simulink model "CL_NL_DH_GUIA"  (R2025b)
settings: Solver=ode4  StartTime=0.0  StopTime=200  FixedStep=Ts  RelTol=1e-3
values from neighbouring files (symbols this model uses):
  att_alt = 0    [guiagem_NL.m]
  h_ref0 = h0    (= 600)    [guiagem_NL.m]
  i = find([Plantas.Ve] == VT_missao & [Plantas.He] == 600, 1)    [guiagem_NL.m]
  K_bank_guia = 0.1975    [guiagem_NL.m]
  phi_max_guia = deg2rad(20)    [guiagem_NL.m]
  phi_psi = 0    [guiagem_NL.m]
  surfaces = 24    [guiagem_NL.m]
  U_trim = double(Plantas(i).Ue(1:4))    [guiagem_NL.m]
  VT_ref0 = VT_missao    [guiagem_NL.m]
  VT_Throttle = 1    [guiagem_NL.m]
  WPs = [ 256    0  600  15 ... (first row only)    [guiagem_NL.m]
undefined symbols (not defined in the file or in its folder): Plantas, R_accept
libraries: simulink_extras x10, simulink x1
settings Model: SimulationMode=accelerator  Creator=mirko  LastModifiedBy=mirko

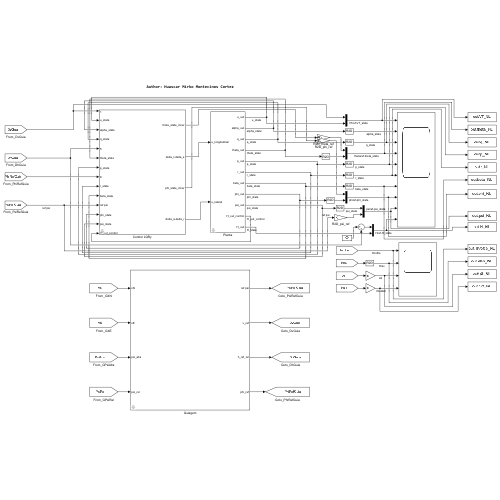
[thumbnail: Simulink's stored preview of the top-level diagram]
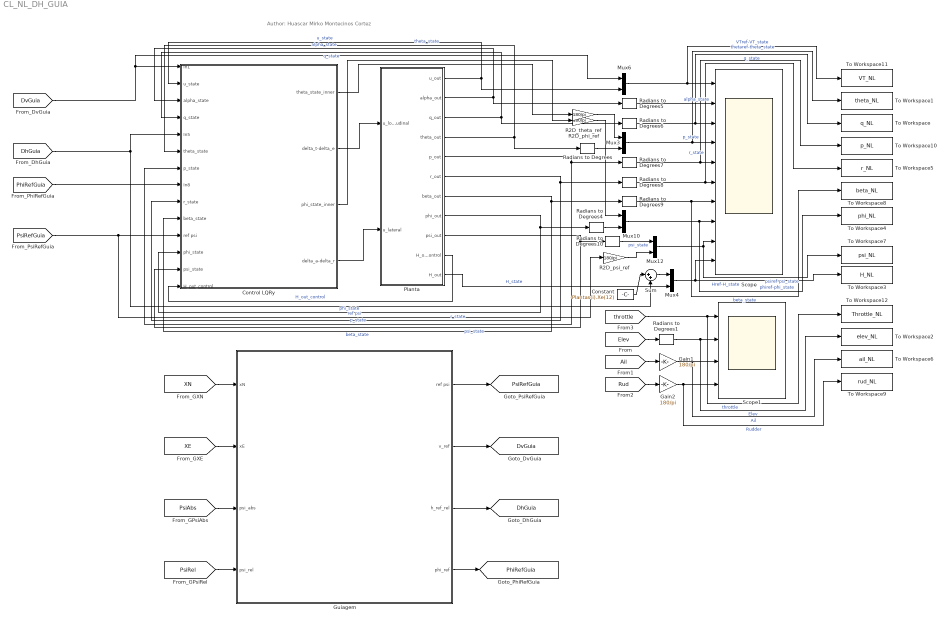
== system CL_NL_DH_GUIA ==
  note: Author: Huascar Mirko Montecinos Cortez
  Constant : Constant  Value=-Plantas(i).Xe(12)
  Control LQRy : Subsystem
  Gain1 : Gain  Gain=180/pi
  Gain2 : Gain  Gain=180/pi
  Guiagem : Subsystem
  Mux{3..4,6,10,12} (5 alike) : Mux  Inputs=2
  Planta : Subsystem
  R2D_phi_ref : Gain  Gain=180/pi
  R2D_psi_ref : Gain  Gain=180/pi
  R2D_theta_ref : Gain  Gain=180/pi
  Radians to Degrees{,1,4..10} (9 alike) : simulink_extras/Transformations/Radians to Degrees
  Scope : Scope  NumInputPorts=10
      settings: ActiveDisplayString=10  ActiveDisplayYMinimum=597.42662245797032  ActiveDisplayYMaximum=600.90765479327524
  Scope1 : Scope  NumInputPorts=4
      settings: ActiveDisplayString=4  ActiveDisplayYMinimum=-5.76866006164083  ActiveDisplayYMaximum=6.0116826932203384
  Sum : Sum  Inputs=|++
  To Workspace : ToWorkspace  VariableName=q_NL  SaveFormat=Structure With Time  SampleTime=-1
  To Workspace1 : ToWorkspace  VariableName=theta_NL  SaveFormat=Structure With Time  SampleTime=-1
  To Workspace10 : ToWorkspace  VariableName=p_NL  SaveFormat=Structure With Time  SampleTime=-1
  To Workspace11 : ToWorkspace  VariableName=VT_NL  SaveFormat=Structure With Time  SampleTime=-1
  To Workspace12 : ToWorkspace  VariableName=Throttle_NL  SaveFormat=Structure With Time  SampleTime=-1
  To Workspace2 : ToWorkspace  VariableName=elev_NL  SaveFormat=Structure With Time  SampleTime=-1
  To Workspace3 : ToWorkspace  VariableName=H_NL  SaveFormat=Structure With Time  SampleTime=-1
  To Workspace4 : ToWorkspace  VariableName=phi_NL  SaveFormat=Structure With Time  SampleTime=-1
  To Workspace5 : ToWorkspace  VariableName=r_NL  SaveFormat=Structure With Time  SampleTime=-1
  To Workspace6 : ToWorkspace  VariableName=ail_NL  SaveFormat=Structure With Time  SampleTime=-1
  To Workspace7 : ToWorkspace  VariableName=psi_NL  SaveFormat=Structure With Time  SampleTime=-1
  To Workspace8 : ToWorkspace  VariableName=beta_NL  SaveFormat=Structure With Time  SampleTime=-1
  To Workspace9 : ToWorkspace  VariableName=rud_NL  SaveFormat=Structure With Time  SampleTime=-1
  tag scope: DhGuia=global, DvGuia=global, PhiRefGuia=global, PsiRefGuia=global
  wires:
  Planta/1(u_out) -> Mux6/2, Control LQRy/2(u_state)  "u_state"
  Planta/2(alpha_out) -> Radians to Degrees5/1, Control LQRy/3(alpha_state)  "alpha_state"
  Planta/3(q_out) -> Radians to Degrees6/1, Control LQRy/4(q_state)  "q_state"
  Planta/4(theta_out) -> Radians to Degrees/1, Control LQRy/6(theta_state)  "theta_state"
  Planta/5(p_out) -> Control LQRy/7(p_state), Radians to Degrees7/1  "p_state"
  Planta/6(r_out) -> Radians to Degrees8/1, Control LQRy/9(r_state)  "r_state"
  Planta/7(beta_out) -> Control LQRy/10(beta_state), Radians to Degrees9/1  "beta_state"
  Planta/8(phi_out) -> Control LQRy/12(phi_state), Radians to Degrees4/1  "phi_state"
  Planta/9(psi_out) -> Control LQRy/13(psi_state), Radians to Degrees10/1  "psi_state"
  Mux3/1 -> To Workspace1/1, Scope/4  "thetaref-theta_state"
  Radians to Degrees/1 -> Mux3/2
  Mux4/1 -> Scope/10, To Workspace3/1  "Href-H_state"
  Constant/1 -> Sum/1
  Sum/1 -> Mux4/1
  Radians to Degrees1/1 -> Scope1/2, To Workspace2/1  "Elev"
  Gain1/1 -> Scope1/3, To Workspace6/1  "Ail"
  Gain2/1 -> Scope1/4, To Workspace9/1  "Rudder"
  [Elev] -> Radians to Degrees1/1
  [Ail] -> Gain1/1
  [Rud] -> Gain2/1
  [throttle] -> To Workspace12/1, Scope1/1  "throttle"
  Mux6/1 -> To Workspace11/1, Scope/1  "VTref-VT_state"
  Mux10/1 -> To Workspace4/1, Scope/8  "phiref-phi_state"
  Radians to Degrees4/1 -> Mux10/2
  Radians to Degrees5/1 -> Scope/2  "alpha_state"
  Radians to Degrees6/1 -> To Workspace/1, Scope/3  "q_state"
  Radians to Degrees7/1 -> To Workspace10/1, Scope/5  "p_state"
  Radians to Degrees8/1 -> Scope/6, To Workspace5/1  "r_state"
  Radians to Degrees9/1 -> Scope/7, To Workspace8/1  "beta_state"
  Mux12/1 -> To Workspace7/1, Scope/9  "psiref-psi_state"
  Planta/11(H_out) -> Mux4/2  "H_state"
  Radians to Degrees10/1 -> Mux12/1  "psi_state"
  [DhGuia] -> Sum/2, Control LQRy/5(In5)
  [DvGuia] -> Mux6/1, Control LQRy/1(In1)
  R2D_theta_ref/1 -> Mux3/1
  R2D_psi_ref/1 -> Mux12/2
  R2D_phi_ref/1 -> Mux10/1
  [PsiRefGuia] -> R2D_psi_ref/1, Control LQRy/11(ref psi)  "ref psi"
  [PhiRefGuia] -> Control LQRy/8(In8)
  Planta/10(H_out_control) -> Control LQRy/14(H_out_control)  "H_out_control"
  Control LQRy/1(theta_state_inner) -> R2D_theta_ref/1
  Control LQRy/2(delta_t-delta_e) -> Planta/1(u_longitudinal)
  Control LQRy/3(phi_state_inner) -> R2D_phi_ref/1
  Control LQRy/4(delta_a-delta_r) -> Planta/2(u_lateral)
  [XN] -> Guiagem/1(xN)
  [XE] -> Guiagem/2(xE)
  [PsiAbs] -> Guiagem/3(psi_abs)
  [PsiRel] -> Guiagem/4(psi_rel)
  Guiagem/1(ref psi) -> [PsiRefGuia]
  Guiagem/2(v_ref) -> [DvGuia]
  Guiagem/3(h_ref_rel) -> [DhGuia]
  Guiagem/4(phi_ref) -> [PhiRefGuia]

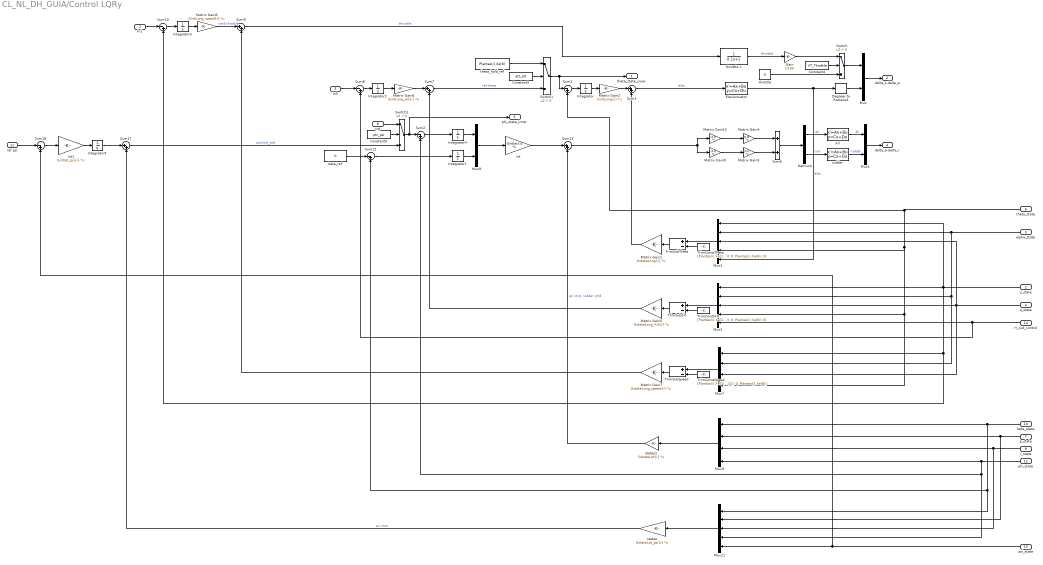
== system CL_NL_DH_GUIA/Control LQRy ==
  In1 : Inport
  u_state : Inport  Port=2
  alpha_state : Inport  Port=3
  q_state : Inport  Port=4
  In5 : Inport  Port=5
  theta_state : Inport  Port=6
  p_state : Inport  Port=7
  In8 : Inport  Port=8
  r_state : Inport  Port=9
  beta_state : Inport  Port=10
  ref psi : Inport  Port=11
  phi_state : Inport  Port=12
  psi_state : Inport  Port=13
  H_out_control : Inport  Port=14
  Ail : StateSpace  A=-surfaces  B=surfaces  D=0  InitialCondition=0
  Constant2 : Constant  Value=VT_Throttle
  Constant3 : Constant  Value=att_alt
  Constant4 : Constant  Value=phi_psi
  Degrees to Radians3 : simulink_extras/Transformations/Degrees to Radians
  Demux4 : Demux  Outputs=2
      settings: DisplayOption=none
  ElevActuator : StateSpace  A=-surfaces  B=surfaces  D=0  InitialCondition=Plantas(i).Ue(2)
  Gain : Gain  Gain=1/100
  Integrator{,1..5} (6 alike) : Integrator
  Matrix Gain1 : Gain  Gain=GstateLong{i}  Multiplication=Matrix(K*u)  SaturateOnIntegerOverflow=on  OutDataTypeStr=Inherit: Same as input  ParamDataTypeStr=Inherit: Same as input
  Matrix Gain10 : Gain  Gain=[1 0]  Multiplication=Matrix(K*u)  SaturateOnIntegerOverflow=on  OutDataTypeStr=Inherit: Same as input  ParamDataTypeStr=Inherit: Same as input
  Matrix Gain2 : Gain  Gain=GintLong{i}  Multiplication=Matrix(K*u)  SaturateOnIntegerOverflow=on  OutDataTypeStr=Inherit: Same as input  ParamDataTypeStr=Inherit: Same as input
  Matrix Gain3 : Gain  Gain=[0 1]'  Multiplication=Matrix(K*u)  SaturateOnIntegerOverflow=on  OutDataTypeStr=Inherit: Same as input  ParamDataTypeStr=Inherit: Same as input
  Matrix Gain4 : Gain  Gain=[1 0]'  Multiplication=Matrix(K*u)  SaturateOnIntegerOverflow=on  OutDataTypeStr=Inherit: Same as input  ParamDataTypeStr=Inherit: Same as input
  Matrix Gain5 : Gain  Gain=GstateLong_Alt{i}  Multiplication=Matrix(K*u)  SaturateOnIntegerOverflow=on  OutDataTypeStr=Inherit: Same as input  ParamDataTypeStr=Inherit: Same as input
  Matrix Gain6 : Gain  Gain=GintLong_Alt{i}  Multiplication=Matrix(K*u)  SaturateOnIntegerOverflow=on  OutDataTypeStr=Inherit: Same as input  ParamDataTypeStr=Inherit: Same as input
  Matrix Gain7 : Gain  Gain=GstateLong_speed{i}  Multiplication=Matrix(K*u)  SaturateOnIntegerOverflow=on  OutDataTypeStr=Inherit: Same as input  ParamDataTypeStr=Inherit: Same as input
  Matrix Gain8 : Gain  Gain=GintLong_speed{i}  Multiplication=Matrix(K*u)  SaturateOnIntegerOverflow=on  OutDataTypeStr=Inherit: Same as input  ParamDataTypeStr=Inherit: Same as input
  Matrix Gain9 : Gain  Gain=[0 1]  Multiplication=Matrix(K*u)  SaturateOnIntegerOverflow=on  OutDataTypeStr=Inherit: Same as input  ParamDataTypeStr=Inherit: Same as input
  Mux : Mux  Inputs=2
  Mux1 : Mux  Inputs=2
  Mux11 : Mux  Inputs=5
  Mux2 : Mux  Inputs=5
  Mux5 : Mux  Inputs=5
  Mux7 : Mux
  Mux8 : Mux  Inputs=2
  Mux9 : Mux
  Sum1 : Sum  Inputs=|-+
  Sum10 : Sum  Inputs=|-+
  Sum12 : Sum  Inputs=|-+  SaturateOnIntegerOverflow=on
  Sum13 : Sum  Inputs=|++  SaturateOnIntegerOverflow=on
  Sum17 : Sum  Inputs=|++  SaturateOnIntegerOverflow=on
  Sum18 : Sum  Inputs=|-+  SaturateOnIntegerOverflow=on
  Sum2 : Sum  Inputs=|-+  SaturateOnIntegerOverflow=on
  Sum3 : Sum  Inputs=|++
  Sum6 : Sum  Inputs=2  SaturateOnIntegerOverflow=on
  Sum7 : Sum  Inputs=|++
  Sum8 : Sum  Inputs=|-+
  Sum9 : Sum  Inputs=|++
  Switch : Switch  Criteria=u2 > Threshold  SaturateOnIntegerOverflow=off  InputSameDT=off
  Switch1 : Switch  Criteria=u2 > Threshold  SaturateOnIntegerOverflow=off  InputSameDT=off
  Switch2 : Switch  Criteria=u2 > Threshold  SaturateOnIntegerOverflow=off  InputSameDT=off
  TrimConstAlt : Constant  Value=[Plantas(i).Xe(1); atan(Plantas(i).Xe(3)/Plantas(i).Xe(1)); 0; Plantas(i).Xe(8); 0]  VectorParams1D=off
  TrimConstSpeed : Constant  Value=[Plantas(i).Xe(1); atan(Plantas(i).Xe(3)/Plantas(i).Xe(1)); 0; Plantas(i).Xe(8)]  VectorParams1D=off
  TrimConstTheta : Constant  Value=[Plantas(i).Xe(1); atan(Plantas(i).Xe(3)/Plantas(i).Xe(1)); 0; Plantas(i).Xe(8); 0]  VectorParams1D=off
  TrimSubAlt : Sum  Inputs=+-
  TrimSubSpeed : Sum  Inputs=+-
  TrimSubTheta : Sum  Inputs=+-
  beta_ref : Constant  Value=0
  int : Gain  Gain=Gintlat{i}  Multiplication=Matrix(K*u)  SaturateOnIntegerOverflow=on  OutDataTypeStr=Inherit: Same as input  ParamDataTypeStr=Inherit: Same as input
  int1 : Gain  Gain=Gintlat_psi{i}  Multiplication=Matrix(K*u)  SaturateOnIntegerOverflow=on  OutDataTypeStr=Inherit: Same as input  ParamDataTypeStr=Inherit: Same as input
  rudder : StateSpace  A=-surfaces  B=surfaces  D=0  InitialCondition=0
  states : Gain  Gain=GstateLat_psi{i}  Multiplication=Matrix(K*u)  SaturateOnIntegerOverflow=on  OutDataTypeStr=Inherit: Same as input  ParamDataTypeStr=Inherit: Same as input
  states1 : Gain  Gain=GstateLat{i}  Multiplication=Matrix(K*u)  SaturateOnIntegerOverflow=on  OutDataTypeStr=Inherit: Same as input  ParamDataTypeStr=Inherit: Same as input
  theta_hold_ref : Constant  Value=Plantas(i).Xe(8)
  throttle : Constant  Value=0
  throttle 1 : TransferFcn  Denominator=[0.1 1]
  theta_state_inner : Outport
  delta_t-delta_e : Outport  Port=2
  phi_state_inner : Outport  Port=3
  delta_a-delta_r : Outport  Port=4
  wires:
  Constant4/1 -> Switch2/2
  Constant3/1 -> Switch1/2
  q_state/1 -> Mux2/3, Mux7/3, Mux5/3
  Matrix Gain6/1 -> Sum7/1
  theta_state/1 -> Mux7/4, Mux5/4, Mux2/4, Sum1/2
  Constant2/1 -> Switch/2
  Mux9/1 -> states1/1
  states1/1 -> Sum13/2  "ail cmd, rudder cmd"
  Mux1/1 -> delta_a-delta_r/1
  Mux5/1 -> TrimSubAlt/1
  Mux2/1 -> TrimSubTheta/1
  Integrator5/1 -> Sum17/1
  alpha_state/1 -> Mux7/2, Mux5/2, Mux2/2
  Sum10/1 -> Integrator3/1
  states/1 -> Sum17/2  "ail cmd"
  r_state/1 -> Mux9/3, Mux11/3
  Demux4/2 -> rudder/1  "rud"
  p_state/1 -> Mux9/2, Mux11/2
  Sum18/1 -> int1/1
  Degrees to Radians3/1 -> Mux/2
  Matrix Gain9/1 -> Matrix Gain3/1
  Sum3/1 -> ElevActuator/1  "elev"
  u_state/1 -> Mux2/1, Mux7/1, Sum10/2, Mux5/1
  TrimConstAlt/1 -> TrimSubAlt/2
  Sum6/1 -> Demux4/1
  Integrator1/1 -> Mux8/2
  psi_state/1 -> Mux11/5, Sum18/2
  TrimSubTheta/1 -> Matrix Gain1/1
  Integrator/1 -> Matrix Gain2/1
  Ail/1 -> Mux1/1  "Ail"
  Sum9/1 -> throttle 1/1  "throttle"
  Integrator3/1 -> Matrix Gain8/1
  beta_ref/1 -> Sum12/1
  Integrator4/1 -> Mux8/1
  Matrix Gain3/1 -> Sum6/2
  Sum13/1 -> Matrix Gain9/1, Matrix Gain10/1
  H_out_control/1 -> Mux5/5, Sum8/2
  Gain/1 -> Switch/1
  ElevActuator/1 -> Degrees to Radians3/1, Mux2/5  "elev"
  Matrix Gain10/1 -> Matrix Gain4/1
  phi_state/1 -> Mux11/4, Sum2/2, Mux9/4
  Sum2/1 -> Integrator4/1
  TrimConstTheta/1 -> TrimSubTheta/2
  Switch2/1 -> phi_state_inner/1, Sum2/1
  throttle 1/1 -> Gain/1  "throttle"
  Matrix Gain2/1 -> Sum3/1
  beta_state/1 -> Mux9/1, Mux11/1, Sum12/2
  Sum8/1 -> Integrator2/1
  Matrix Gain5/1 -> Sum7/2
  Switch1/1 -> theta_state_inner/1, Sum1/1
  Sum17/1 -> Switch2/3  "psiCmd_rad"
  Matrix Gain8/1 -> Sum9/1  "cmd throttle"
  TrimSubAlt/1 -> Matrix Gain5/1
  Sum12/1 -> Integrator1/1
  Integrator2/1 -> Matrix Gain6/1
  In5/1 -> Sum8/1
  TrimSubSpeed/1 -> Matrix Gain7/1
  Sum7/1 -> Switch1/3  "ref theta"
  throttle/1 -> Switch/3
  int1/1 -> Integrator5/1
  Mux8/1 -> int/1
  Mux11/1 -> states/1
  Mux7/1 -> TrimSubSpeed/1
  rudder/1 -> Mux1/2  "rudder"
  Mux/1 -> delta_t-delta_e/1
  int/1 -> Sum13/1
  Matrix Gain4/1 -> Sum6/1
  Switch/1 -> Mux/1
  Sum1/1 -> Integrator/1
  theta_hold_ref/1 -> Switch1/1
  Matrix Gain1/1 -> Sum3/2
  Matrix Gain7/1 -> Sum9/2
  Demux4/1 -> Ail/1  "ail"
  TrimConstSpeed/1 -> TrimSubSpeed/2
  In1/1 -> Sum10/1
  In8/1 -> Switch2/1
  ref psi/1 -> Sum18/1

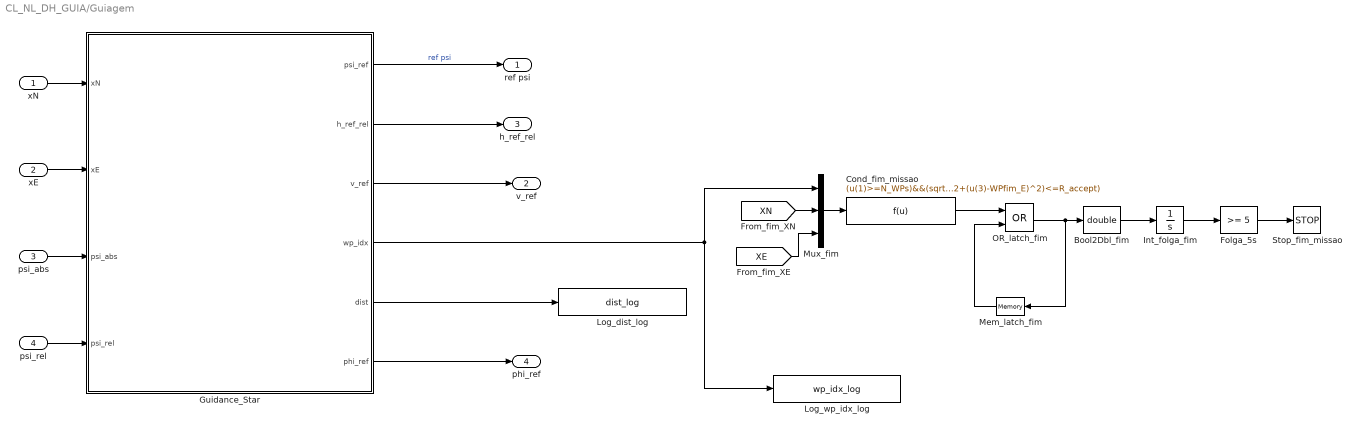
== system CL_NL_DH_GUIA/Guiagem ==
  xN : Inport
  xE : Inport  Port=2
  psi_abs : Inport  Port=3
  psi_rel : Inport  Port=4
  Bool2Dbl_fim : DataTypeConversion  OutDataTypeStr=double  SaturateOnIntegerOverflow=off  RndMeth=Floor
  Cond_fim_missao : Fcn  Expr=(u(1)>=N_WPs)&&(sqrt((u(2)-WPfim_N)^2+(u(3)-WPfim_E)^2)<=R_accept)
  Folga_5s : simulink/Logic and Bit Operations/Compare To Constant  relop=>=  const=5  OutDataTypeStr=boolean
  Guidance_Star : MATLAB Function  TreatAsAtomicUnit=on
  Int_folga_fim : Integrator
  Log_dist_log : ToWorkspace  VariableName=dist_log  SampleTime=-1
  Log_wp_idx_log : ToWorkspace  VariableName=wp_idx_log  SampleTime=-1
  Mem_latch_fim : Memory
  Mux_fim : Mux  Inputs=3
  OR_latch_fim : Logic  Operator=OR  AllPortsSameDT=off  OutDataTypeStr=boolean
  Stop_fim_missao : Stop
  ref psi : Outport
  v_ref : Outport  Port=2
  h_ref_rel : Outport  Port=3
  phi_ref : Outport  Port=4
  wires:
  Mem_latch_fim/1 -> OR_latch_fim/2
  [XN] -> Mux_fim/2
  Guidance_Star/6(phi_ref) -> phi_ref/1
  Guidance_Star/5(dist) -> Log_dist_log/1
  Int_folga_fim/1 -> Folga_5s/1
  Mux_fim/1 -> Cond_fim_missao/1
  [XE] -> Mux_fim/3
  Cond_fim_missao/1 -> OR_latch_fim/1
  xN/1 -> Guidance_Star/1(xN)
  Folga_5s/1 -> Stop_fim_missao/1
  Bool2Dbl_fim/1 -> Int_folga_fim/1
  Guidance_Star/4(wp_idx) -> Log_wp_idx_log/1, Mux_fim/1
  OR_latch_fim/1 -> Mem_latch_fim/1, Bool2Dbl_fim/1
  Guidance_Star/1(psi_ref) -> ref psi/1  "ref psi"
  psi_rel/1 -> Guidance_Star/4(psi_rel)
  psi_abs/1 -> Guidance_Star/3(psi_abs)
  Guidance_Star/3(v_ref) -> v_ref/1
  Guidance_Star/2(h_ref_rel) -> h_ref_rel/1
  xE/1 -> Guidance_Star/2(xE)

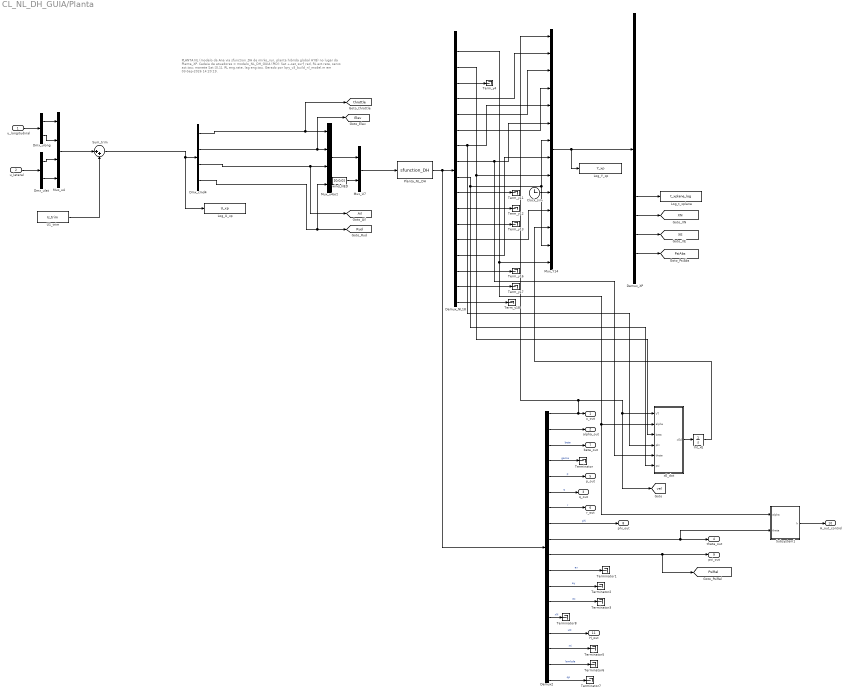
== system CL_NL_DH_GUIA/Planta ==
  note: PLANTA NL (modelo da Ana via sfunction_DH de mirko_run, planta hibrida global HYB)
      | no lugar da Planta_XP. Cadeia de atuadores = modelo_NL_DH_GUIA (PID): Sat +-sat_surf_rad, RL act.rate,
      | servo act.tau; manete Sat [0,1], RL eng.rate, lag eng.tau. Gerado por lqry_v3_build_nl_model.m em 03-Sep-2026 14:20:19.
  u_longitudinal : Inport
  u_lateral : Inport  Port=2
  Clock_sim : Clock
  Demux2 : Demux  Outputs=18
  Demux_NL18 : Demux  Outputs=18
  Demux_XP : Demux  Outputs=14
  Dmx_cmd4 : Demux
  Dmx_ulat : Demux  Outputs=2
  Dmx_ulong : Demux  Outputs=2
  Int_xE : Integrator
  Log_U_xp : ToWorkspace  VariableName=U_xp  SampleTime=-1
  Log_Y_xp : ToWorkspace  VariableName=Y_xp  SampleTime=-1
  Log_t_xplane : ToWorkspace  VariableName=t_xplane_log  SampleTime=-1
  Mux_U7 : Mux  Inputs=2
  Mux_Y14 : Mux  Inputs=14
  Mux_u4 : Mux
  Mux_u4act : Mux
  Planta_NL_DH : S-Function  FunctionName=sfunction_DH  Parameters=Xe_planta, coef_Sato, coef_Ana, Variacao_Iner  SFunctionDeploymentMode=off  EnableBusSupport=off
  Subsystem1 : Subsystem
  Sum_trim : Sum  Inputs=|++
  Term_y{4,11..13,16..18} (7 alike) : Terminator
  Terminator{,1..3,5..8} (8 alike) : Terminator
  U1_trim : Constant  Value=U_trim
  wind_NED : Constant  Value=[0;0;0]
  xE_dot : MATLAB Function  TreatAsAtomicUnit=on
  u_out : Outport
  alpha_out : Outport  Port=2
  q_out : Outport  Port=3
  theta_out : Outport  Port=4
  p_out : Outport  Port=5
  r_out : Outport  Port=6
  beta_out : Outport  Port=7
  phi_out : Outport  Port=8
  psi_out : Outport  Port=9
  H_out_control : Outport  Port=10
  H_out : Outport  Port=11
  tag scope: Ail=global, Elev=global, PsiAbs=global, PsiRel=global, Rud=global, XE=global, XN=global, throttle=global, vel=global
  wires:
  u_longitudinal/1 -> Dmx_ulong/1
  u_lateral/1 -> Dmx_ulat/1
  Dmx_ulong/1 -> Mux_u4/1
  Dmx_ulong/2 -> Mux_u4/2
  Dmx_ulat/1 -> Mux_u4/3
  Dmx_ulat/2 -> Mux_u4/4
  Demux2/2 -> alpha_out/1
  Demux2/9 -> Subsystem1/2(theta), theta_out/1
  Demux2/10 -> [PsiRel], psi_out/1
  Subsystem1/1(h) -> H_out_control/1
  Demux_XP/11 -> [XN]
  Demux_XP/12 -> [XE]
  Demux_XP/13 -> [PsiAbs]
  Demux_XP/10 -> Log_t_xplane/1
  Mux_u4/1 -> Sum_trim/1
  U1_trim/1 -> Sum_trim/2
  Sum_trim/1 -> Dmx_cmd4/1, Log_U_xp/1
  Dmx_cmd4/1 -> [throttle], Mux_u4act/1
  Dmx_cmd4/2 -> [Elev], Mux_u4act/2
  Dmx_cmd4/3 -> [Ail], Mux_u4act/3
  Dmx_cmd4/4 -> [Rud], Mux_u4act/4
  Mux_u4act/1 -> Mux_U7/1
  wind_NED/1 -> Mux_U7/2
  Mux_U7/1 -> Planta_NL_DH/1
  Planta_NL_DH/1 -> Demux2/1, Demux_NL18/1
  Demux_NL18/4 -> Term_y4/1
  Demux_NL18/11 -> Term_y11/1
  Demux_NL18/12 -> Term_y12/1
  Demux_NL18/13 -> Term_y13/1
  Demux_NL18/16 -> Term_y16/1
  Demux_NL18/17 -> Term_y17/1
  Demux_NL18/18 -> Term_y18/1
  Demux2/1 -> [vel], xE_dot/1(VT), Mux_Y14/1, u_out/1
  Demux_NL18/2 -> Subsystem1/1(alpha), xE_dot/2(alpha), Mux_Y14/14
  Demux_NL18/3 -> xE_dot/3(beta), Mux_Y14/9
  Demux_NL18/8 -> Mux_Y14/5, xE_dot/4(phi)
  Demux_NL18/9 -> xE_dot/5(theta), Mux_Y14/6
  Demux_NL18/10 -> Mux_Y14/7, Mux_Y14/13, xE_dot/6(psi)
  xE_dot/1(xEd) -> Int_xE/1
  Demux_NL18/5 -> Mux_Y14/2
  Demux_NL18/6 -> Mux_Y14/3
  Demux_NL18/7 -> Mux_Y14/4
  Demux_NL18/15 -> Mux_Y14/8
  Clock_sim/1 -> Mux_Y14/10
  Demux_NL18/14 -> Mux_Y14/11
  Int_xE/1 -> Mux_Y14/12
  Mux_Y14/1 -> Log_Y_xp/1, Demux_XP/1
  Demux2/3 -> beta_out/1  "beta"
  Demux2/4 -> Terminator/1  "gama"
  Demux2/6 -> q_out/1  "q"
  Demux2/5 -> p_out/1  "p"
  Demux2/7 -> r_out/1  "r"
  Demux2/8 -> phi_out/1  "phi"
  Demux2/15 -> H_out/1  "xD"
  Demux2/11 -> Terminator1/1  "ax"
  Demux2/12 -> Terminator2/1  "ay"
  Demux2/13 -> Terminator3/1  "az"
  Demux2/16 -> Terminator5/1  "mi"
  Demux2/17 -> Terminator6/1  "lambda"
  Demux2/18 -> Terminator7/1  "qp"
  Demux2/14 -> Terminator8/1  "xN"

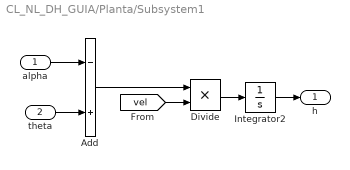
== system CL_NL_DH_GUIA/Planta/Subsystem1 ==
  alpha : Inport
  theta : Inport  Port=2
  Add : Sum  Inputs=-+
  Divide : Product  Inputs=**
  Integrator2 : Integrator
  h : Outport
  wires:
  Add/1 -> Divide/1
  Integrator2/1 -> h/1
  Divide/1 -> Integrator2/1
  alpha/1 -> Add/1
  theta/1 -> Add/2
  [vel] -> Divide/2

== matlab function CL_NL_DH_GUIA/Planta/xE_dot ==
  data: VT input; xEd output; alpha input; beta input; phi input; theta input; psi input
function xEd = xE_dot(VT, alpha, beta, phi, theta, psi)
% velocidade Leste inercial reconstruida das saidas do observador
% (exato p/ vento zero): [u v w] do triedro aerodinamico -> Lnb linha 2.
u = VT*cos(alpha)*cos(beta); v = VT*sin(beta); w = VT*sin(alpha)*cos(beta);
xEd = (sin(phi)*sin(theta)*sin(psi)+cos(phi)*cos(psi))*v ...
    + (cos(phi)*sin(theta)*sin(psi)-sin(phi)*cos(psi))*w ...
    + cos(theta)*sin(psi)*u;
end

== matlab function CL_NL_DH_GUIA/Guiagem/Guidance_Star ==
  settings: updateMethod=DISCRETE  sampleTime=0.05
  data: xN input; psi_ref output; xE input; psi_abs input; psi_rel input; h_ref_rel output; v_ref output; wp_idx output; dist output; phi_ref output; WPs parameter; R_accept parameter; h_ref0 parameter; VT_ref0 parameter; K_bank_guia parameter; phi_max_guia parameter
function [psi_ref, h_ref_rel, v_ref, wp_idx, dist, phi_ref] = Guidance_Star(xN, xE, psi_abs, psi_rel, WPs, R_accept, h_ref0, VT_ref0, K_bank_guia, phi_max_guia)
% Guiagem LOS por waypoints (algoritmo do PIPER-1-6 do Julio, adaptado ao DH).
% Entradas: posicao xN/xE [m], proa absoluta psi_abs e relativa ao engate psi_rel [rad].
% WPs = [N E h V] (uma linha por waypoint); R_accept = raio de captura [m].
% Saidas (entram DIRETO nos holds do LQRy):
%   psi_ref   [rad] proa de referencia no mesmo referencial (relativo ao engate) que o psi Hold realimenta
%   h_ref_rel [m]   altitude do WP - h_ref0 (o Alt Hold trabalha com H relativa ao engate)
%   v_ref     [m/s] velocidade do WP (absoluta) -> Vel Hold
%   phi_ref   [rad] bank-to-turn, so' usado no modo phi Hold (phi_psi = 1); zero apos o ultimo WP
%   wp_idx, dist: monitor (WP alvo e distancia ate ele)
persistent k hold_fim
if isempty(k), k = 1; 
    hold_fim = 0; 
end
n = size(WPs, 1); 
if k > n, k = n;
end

dist = sqrt((WPs(k,1) - xN)^2 + (WPs(k,2) - xE)^2);

if dist <= R_accept
    if k < n, k = k + 1; else, hold_fim = 1; end
end

psi_los = atan2(WPs(k,2) - xE, WPs(k,1) - xN);

dpsi = mod(psi_los - psi_abs + pi, 2*pi) - pi;

psi_ref = psi_rel + dpsi;

if hold_fim, phi_ref = 0; else, phi_ref = min(max(K_bank_guia*dpsi, -phi_max_guia), phi_max_guia); end
h_ref_rel = WPs(k,3) - h_ref0;
v_ref = WPs(k,4) + 0*VT_ref0;
wp_idx = k;
end
